simulink model "FirstOrderSMC"  (R2015b)
settings: Solver=VariableStepAuto  StartTime=0.0  StopTime=10.0  RelTol=1e-3
values from neighbouring files (symbols this model uses):
  B = 5    [SMC_Mass_Spring_Damper.m]
  K = 2    [SMC_Mass_Spring_Damper.m]
  M = 2    [SMC_Mass_Spring_Damper.m]
settings Model: Creator=mathi  LastModifiedBy=mathi

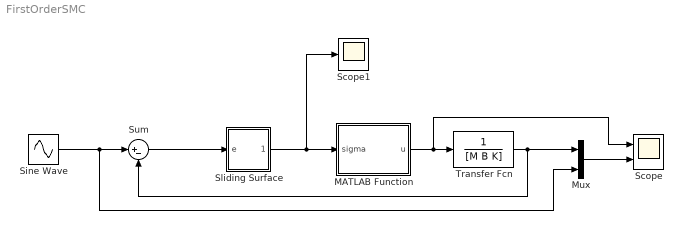
== system FirstOrderSMC ==
  MATLAB Function : MATLAB Function  TreatAsAtomicUnit=on
  Mux : Mux  Inputs=2
  Scope : Scope  NumInputPorts=2
  Scope1 : Scope
  Sine Wave : Sin  Frequency=2  SampleTime=0
  "Sliding Surface " : Subsystem
  Sum : Sum  Inputs=|+-
  Transfer Fcn : TransferFcn  Denominator=[M B K]
  wires:
  Sine Wave/1 -> Mux/2, Sum/1
  Sum/1 -> "Sliding Surface "/1(e)
  Transfer Fcn/1 -> Mux/1, Sum/2
  MATLAB Function/1(u) -> Scope/1, Transfer Fcn/1
  "Sliding Surface "/1(Sigma) -> Scope1/1, MATLAB Function/1(sigma)
  Mux/1 -> Scope/2

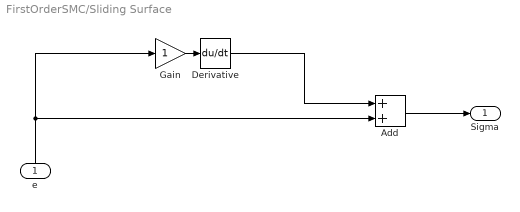
== system FirstOrderSMC/Sliding Surface  ==
  e : Inport
  Add : Sum
  Derivative : Derivative
  Gain : Gain
  Sigma : Outport
  wires:
  Gain/1 -> Derivative/1
  Derivative/1 -> Add/1
  Add/1 -> Sigma/1
  e/1 -> Add/2, Gain/1

== matlab function FirstOrderSMC/MATLAB Function ==
  data: u output; sigma input
function u = fcn(sigma)

u = 20*sign(sigma);
